simulink model "ne_vernoe_vekt_PWM"  (R2019a)
settings: Solver=ode8  StartTime=0.0  StopTime=2  FixedStep=1e-5  RelTol=1e-3
libraries: powerlib x10, powerlib_meascontrol x5
settings Model: Creator=Sozonov_AA  LastModifiedBy=Sozonov_AA

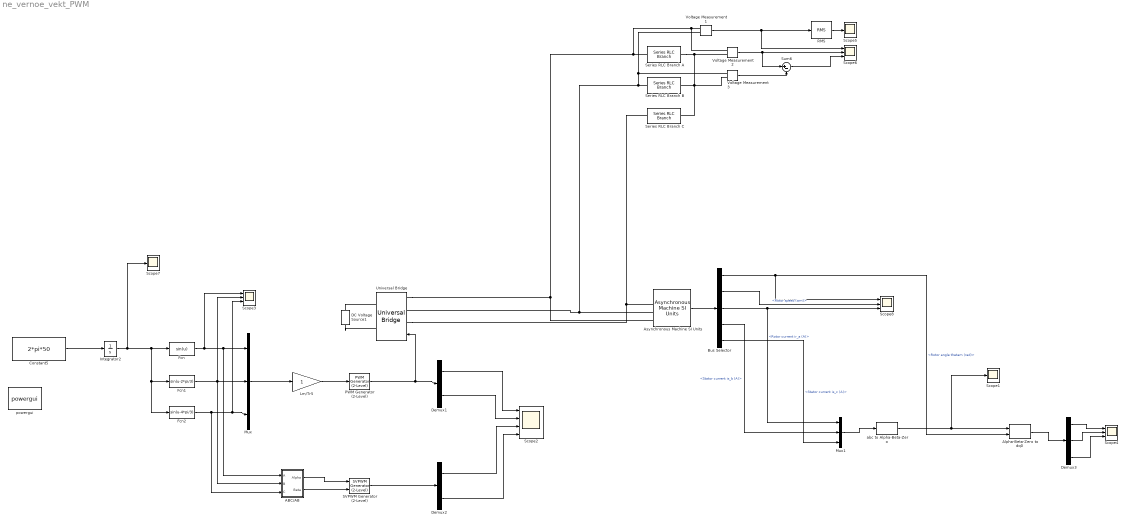
== system ne_vernoe_vekt_PWM ==
  ABC/AB : Subsystem
  Alpha-Beta-Zero to dq0 : powerlib_meascontrol/Transformations/Alpha-Beta-Zero to dq0  Alignment=90 degrees behind phase A axis
      settings: SourceProductName=Simscape Electrical
  Asynchronous Machine SI Units : powerlib/Machines/Asynchronous Machine SI Units  RotorType=Squirrel-cage  PresetModel="16:  10 HP (7.5KW)  400 V 50Hz 1440 RPM"  MechanicalLoad=Torque Tm  ShowDetailedParameters=on  ReferenceFrame=Rotor  Units=SI  MeasurementBus=off  NominalParameters=[7500 400 50]  Stator=[0.7384 0.003045]  Rotor=[0.7402 0.003045]  Cage1=[0.4155 0.002066]  Cage2=[0.4168 0.0003495]  Lm=0.1241  Mechanical=[0.0343 0.000503 2]  PolePairs=2  InitialConditions=[1 0 0 0 0 0 0 0]  SimulateSaturation=off  Saturation=[14.03593122, 27.81365428, 53.79336849, 72.68890987, 97.98006896, 148.6815601, 215.7428561, 302.9841135, 428.7778367 ; 230, 322, 414, 460, 506, 552, 598, 644, 690]  LoadFlowParameters=1492000  TsPowergui=0  TsBlock=-1  IterativeModel=Trapezoidal non iterative  IterativeDiscreteModel=Trapezoidal non iterative  Pmec=1.492e+006
      settings: SourceProductName=Simscape Electrical
  Bus Selector : BusSelector  OutputSignals=Mechanical.Rotor angle thetam (rad),Mechanical.Rotor speed (wm),Rotor measurements.Rotor current ir_a (A),Stator measurements.Stator current is_b (A),Stator measurements.Stator current is_c (A)
  Constant5 : Constant  Value=2*pi*50
  DC Voltage Source1 : powerlib/Electrical Sources/DC Voltage Source  Amplitude=500  Measurements=None
      settings: SourceProductName=Simscape Electrical
  Demux1 : Demux  Outputs=2
  Demux2 : Demux  Outputs=2
  Demux3 : Demux  Outputs=3
  Fcn : Fcn  Expr=sin(u)
  Fcn1 : Fcn  Expr=sin(u-2*pi/3)
  Fcn2 : Fcn  Expr=sin(u-4*pi/3)
  Integrator2 : Integrator  UpperSaturationLimit=2*pi  LowerSaturationLimit=0  WrapState=on  WrappedStateUpperValue=2*pi  WrappedStateLowerValue=0  ZeroCross=off
  Lm/Tr5 : Gain
  Mux : Mux  Inputs=3
  Mux1 : Mux  Inputs=3
  PWM Generator (2-Level) : powerlib_meascontrol/Pulse & Signal Generators/PWM Generator (2-Level)  ModulatorType=Three-phase bridge (6 pulses)  ModulatorMode=Unsynchronized  Fc=2250  Pc=0  nF=27  MinMax=[ -1 1 ]  SamplingTechnique=Natural  ModulatingSignals=off  m=0.8  Freq=60  Phase=0  Ts=0.0001  ShowCarrierOutport=off
  RMS : powerlib_meascontrol/Measurements/RMS  TrueRMS=on  Freq=50  RMSInit=0  Ts=0
      settings: SourceProductName=Simscape Electrical
  SVPWM Generator (2-Level) : powerlib_meascontrol/Pulse & Signal Generators/SVPWM Generator (2-Level)  InputType=alpha-beta components  SwitchingPattern=Pattern #2  Fc=1000  ParUref=[0.8 -30 50]  Ts=0
      settings: SourceProductName=Simscape Electrical  SourceProductBaseCode=PS
  Scope1 : Scope
  Scope2 : Scope  NumInputPorts=4
  Scope{3..4,6,8} (4 alike) : Scope  NumInputPorts=3
  Scope5 : Scope
  Scope7 : Scope
  Series RLC Branch A : powerlib/Elements/Series RLC Branch  LConnTagsString=__new0  RConnTagsString=__new0  BranchType=RL  Resistance=1  Inductance=1/314  SetiL0=off  InitialCurrent=0  Capacitance=1e-6  Setx0=off  InitialVoltage=0  Measurements=Branch voltage and current
      settings: SourceProductName=Simscape Electrical
  Series RLC Branch B : powerlib/Elements/Series RLC Branch  LConnTagsString=__new0  RConnTagsString=__new0  BranchType=RL  Resistance=1  Inductance=1/314  SetiL0=off  InitialCurrent=0  Capacitance=1e-6  Setx0=off  InitialVoltage=0  Measurements=Branch voltage and current
      settings: SourceProductName=Simscape Electrical
  Series RLC Branch C : powerlib/Elements/Series RLC Branch  LConnTagsString=__new0  RConnTagsString=__new0  BranchType=RL  Resistance=1  Inductance=1/314  SetiL0=off  InitialCurrent=0  Capacitance=1e-6  Setx0=off  InitialVoltage=0  Measurements=Branch voltage and current
      settings: SourceProductName=Simscape Electrical
  Sum6 : Sum  Inputs=|+-
  Universal Bridge : powerlib/Power Electronics/Universal Bridge  Arms=3  SnubberResistance=1e5  SnubberCapacitance=inf  Device=IGBT / Diodes  Ron=1e-3  Lon=0  ForwardVoltages="[  0  0  ]"  ForwardVoltage=0  GTOparameters=[ 10e-6 , 20e-6 ]  IGBTparameters=[ 1e-6 , 2e-6 ]  Measurements=None  Measurements_2=None  converterType=Rectifier
      settings: SourceProductName=Simscape Electrical
  Voltage Measurement1 : powerlib/Measurements/Voltage Measurement  PhasorSimulation=off  OutputType=Complex  PSBequivalent=0
      settings: SourceProductName=Simscape Electrical
  Voltage Measurement2 : powerlib/Measurements/Voltage Measurement  PhasorSimulation=off  OutputType=Complex  PSBequivalent=0
      settings: SourceProductName=Simscape Electrical
  Voltage Measurement3 : powerlib/Measurements/Voltage Measurement  PhasorSimulation=off  OutputType=Complex  PSBequivalent=0
      settings: SourceProductName=Simscape Electrical
  abc to Alpha-Beta-Zero : powerlib_meascontrol/Transformations/abc to Alpha-Beta-Zero
      settings: SourceProductName=Simscape Electrical
  powergui : powerlib/powergui  Priority=1  SimulationMode=Continuous  SampleTime=50e-6  frequency=60  Iterations=50  frequencyindice=0  Pbase=100e6  ErrMax=1e-4  UnitsV=kV  UnitsW=MW  buscounter=0  FunctionMessages=off  echomessages=off  EnableUseOfTLC=off  CurrentSourceSwitches=off  DisableSnubberDevices=off  DisableRonSwitches=off  DisableVfSwitches=off  DisplayEquations=off  AutomaticDiscreteSolvers=off  SolverType=Tustin/Backward Euler (TBE)  Interpol=off  ExternalGateDelay=off  methode=off  Ts=100  x0status=blocks  SPID=on  SwTol=0  HookPort=off  NonlinearTolerance=0  nMaxIteration=15  ContinueOnMaxIteration=off  RestoreLinks=warning  ResistiveCurrentMeasurement=off  Frange=[0:2:500]  Ylog=off  Xlog=on  ShowGrid=off  save=off  variable=ZData  structure=0  ZoomFFT=off  StartTime=0.0  cycles=1  DisplayStyle=1  fundamental=60  FreqAxis=off  MaxFrequency=1000  frequencyindicesteady=1  RmsSteady=1  display=off
      settings: SourceProductName=Simscape Electrical
  wires:
  Fcn1/1 -> Scope3/2, Mux/2, ABC/AB/2(B)
  Fcn/1 -> Mux/1, ABC/AB/1(A), Scope3/1
  Constant5/1 -> Integrator2/1
  Integrator2/1 -> Scope7/1, Fcn2/1, Fcn1/1, Fcn/1
  Fcn2/1 -> Mux/3, Scope3/3, ABC/AB/3(C)
  Demux1/1 -> Scope2/1
  Voltage Measurement1/1 -> RMS/1, Scope6/1
  Voltage Measurement2/1 -> Sum6/1, Scope6/2
  Voltage Measurement3/1 -> Sum6/2
  Sum6/1 -> Scope6/3
  RMS/1 -> Scope5/1
  Mux/1 -> Lm/Tr5/1
  Lm/Tr5/1 -> PWM Generator (2-Level)/1
  ABC/AB/1(Alpha) -> SVPWM Generator (2-Level)/1
  ABC/AB/2(Beta) -> SVPWM Generator (2-Level)/2
  SVPWM Generator (2-Level)/1 -> Demux2/1
  PWM Generator (2-Level)/1 -> Universal Bridge/1, Demux1/1
  Demux2/1 -> Scope2/3
  Demux1/2 -> Scope2/2
  Demux2/2 -> Scope2/4
  Alpha-Beta-Zero to dq0/1 -> Demux3/1
  Demux3/1 -> Scope4/1
  Demux3/2 -> Scope4/2
  Demux3/3 -> Scope4/3
  abc to Alpha-Beta-Zero/1 -> Scope1/1, Alpha-Beta-Zero to dq0/1
  Mux1/1 -> abc to Alpha-Beta-Zero/1
  Asynchronous Machine SI Units/1 -> Bus Selector/1
  Bus Selector/2 -> Scope8/2  "<Rotor speed (wm)>"
  Bus Selector/1 -> Scope8/1, Alpha-Beta-Zero to dq0/2  "<Rotor angle thetam (rad)>"
  Bus Selector/3 -> Mux1/1, Scope8/3  "<Rotor current ir_a (A)>"
  Bus Selector/4 -> Mux1/2  "<Stator current is_b (A)>"
  Bus Selector/5 -> Mux1/3  "<Stator current is_c (A)>"
  connections:
  DC Voltage Source1/LConn1 -- Universal Bridge/RConn2
  DC Voltage Source1/RConn1 -- Universal Bridge/RConn1
  Voltage Measurement3/LConn1 -- Voltage Measurement1/LConn2 -- Series RLC Branch B/LConn1 -- Universal Bridge/LConn2 -- Asynchronous Machine SI Units/LConn2
  Universal Bridge/LConn3 -- Voltage Measurement2/LConn1 -- Voltage Measurement1/LConn1 -- Series RLC Branch A/LConn1 -- Asynchronous Machine SI Units/LConn3
  Universal Bridge/LConn1 -- Series RLC Branch C/LConn1 -- Asynchronous Machine SI Units/LConn1
  Series RLC Branch B/RConn1 -- Voltage Measurement2/LConn2 -- Series RLC Branch A/RConn1 -- Voltage Measurement3/LConn2 -- Series RLC Branch C/RConn1

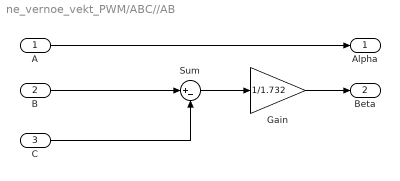
== system ne_vernoe_vekt_PWM/ABC//AB ==
  A : Inport
  B : Inport  Port=2
  C : Inport  Port=3
  Gain : Gain  Gain=1/1.732
  Sum : Sum  Inputs=|+-
  Alpha : Outport
  Beta : Outport  Port=2
  wires:
  B/1 -> Sum/1
  C/1 -> Sum/2
  Sum/1 -> Gain/1
  A/1 -> Alpha/1
  Gain/1 -> Beta/1
